simulink model "IIAFunction"  (R2024b)
settings: Solver=VariableStepAuto  StartTime=0.0  StopTime=80.0  MaxStep=0.01  RelTol=1e-3
values from neighbouring files (symbols this model uses):
  a = 2    [IIAF.m]
  Ac = 2    [IIAF.m]
  b = 2    [IIAF.m]
  Cs = 100    [IIAF.m]
  S0 = 2    [IIAF.m]
  T = 1.5    [IIAF.m]
libraries: SignalEditorBlockLib x2
settings Model: Creator=mefat  LastModifiedBy=mefat

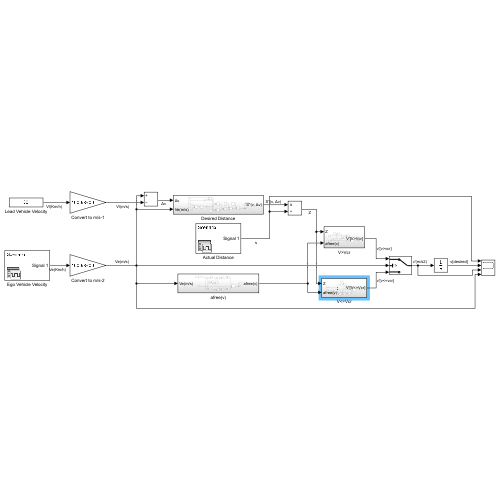
[thumbnail: Simulink's stored preview of the top-level diagram]
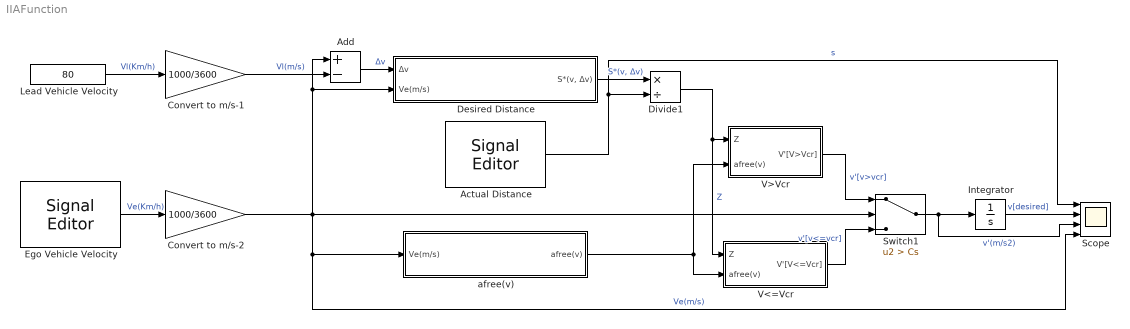
== system IIAFunction ==
  Actual Distance : SignalEditorBlockLib/Signal Editor  FileName=actual_distance.mat  ActiveScenario=Scenario  ActiveSignal=Signal 1  IsBus=off  OutputBusObjectStr=Bus: BusObject  SampleTime=0  ZeroCross=off  OutputAfterFinalValue=Setting to zero  Unit=m  PreserveSignalName=on  ApplySigPropsToAllScenarios=on  ApplySigPropsToAllSignals=off
  Add : Sum  Inputs=+-
  Convert to m/s-1 : Gain  Gain=1000/3600
  Convert to m/s-2 : Gain  Gain=1000/3600
  Desired Distance : Subsystem
  Divide1 : Product  Inputs=*/
  Ego Vehicle Velocity : SignalEditorBlockLib/Signal Editor  FileName=ego_vehicle_velocity.mat  ActiveScenario=Scenario  ActiveSignal=Signal 1  IsBus=off  OutputBusObjectStr=Bus: BusObject  SampleTime=0  ZeroCross=off  OutputAfterFinalValue=Setting to zero  Unit=m/s  PreserveSignalName=on  ApplySigPropsToAllScenarios=on  ApplySigPropsToAllSignals=off
  Integrator : Integrator
  Lead Vehicle Velocity : Constant  Value=80
  Scope : Scope  NumInputPorts=4
  Switch1 : Switch  Criteria=u2 > Threshold  Threshold=Cs  SaturateOnIntegerOverflow=off  InputSameDT=off
  V<=Vcr : Subsystem
  V>Vcr : Subsystem
  afree(v) : Subsystem
  wires:
  Convert to m/s-2/1 -> Scope/4, afree(v)/1(Ve(m/s)), Switch1/2, Add/1, Desired Distance/2(Ve(m/s))  "Ve(m/s)"
  Actual Distance/1 -> Divide1/2, Scope/1  "s"
  Ego Vehicle Velocity/1 -> Convert to m/s-2/1  "Ve(Km/h)"
  Divide1/1 -> V>Vcr/1(Z), V<=Vcr/1(Z)  "Z"
  Desired Distance/1("S*(v, Δv)") -> Divide1/1  "S*(v, Δv)"
  Lead Vehicle Velocity/1 -> Convert to m/s-1/1  "Vl(Km/h)"
  V<=Vcr/1(V'[V<=Vcr]) -> Switch1/3  "v'[v<=vcr]"
  V>Vcr/1(V'[V>Vcr]) -> Switch1/1  "v'[v>vcr]"
  Switch1/1 -> Scope/3, Integrator/1  "v'(m/s2)"
  afree(v)/1(afree(v)) -> V<=Vcr/2(afree(v)), V>Vcr/2(afree(v))
  Integrator/1 -> Scope/2  "v[desired]"
  Add/1 -> Desired Distance/1(Δv)  "Δv"
  Convert to m/s-1/1 -> Add/2  "Vl(m/s)"

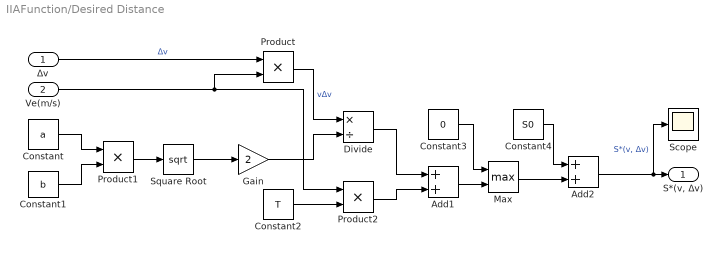
== system IIAFunction/Desired Distance ==
  Δv : Inport
  Ve(m/s) : Inport  Port=2
  Add1 : Sum
  Add2 : Sum
  Constant : Constant  Value=a
  Constant1 : Constant  Value=b
  Constant2 : Constant  Value=T
  Constant3 : Constant  Value=0
  Constant4 : Constant  Value=S0
  Divide : Product  Inputs=*/
  Gain : Gain  Gain=2
  Max : MinMax  Function=max  Inputs=2
  Product : Product
  Product1 : Product
  Product2 : Product
  Scope : Scope
  Square Root : Sqrt
  "S*(v, Δv)" : Outport
  wires:
  Constant/1 -> Product1/1
  Constant2/1 -> Product2/2
  Constant1/1 -> Product1/2
  Square Root/1 -> Gain/1
  Product1/1 -> Square Root/1
  Product2/1 -> Add1/2
  Gain/1 -> Divide/2
  Max/1 -> Add2/2
  Add1/1 -> Max/2
  Add2/1 -> Scope/1, "S*(v, Δv)"/1  "S*(v, Δv)"
  Δv/1 -> Product/1  "Δv"
  Constant4/1 -> Add2/1
  Divide/1 -> Add1/1
  Ve(m/s)/1 -> Product/2, Product2/1
  Constant3/1 -> Max/1
  Product/1 -> Divide/1  "vΔv"

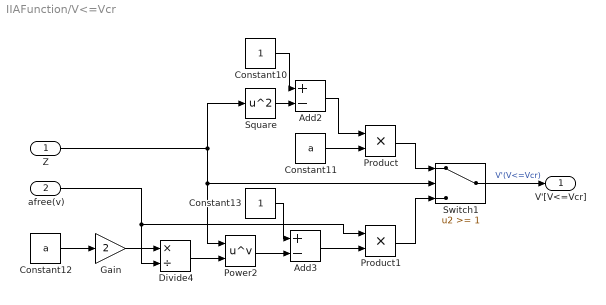
== system IIAFunction/V<=Vcr ==
  Z : Inport
  afree(v) : Inport  Port=2
  Add2 : Sum  Inputs=+-
  Add3 : Sum  Inputs=+-
  Constant10 : Constant
  Constant11 : Constant  Value=a
  Constant12 : Constant  Value=a
  Constant13 : Constant
  Divide4 : Product  Inputs=*/
  Gain : Gain  Gain=2
  Power2 : Math  Operator=pow
  Product : Product
  Product1 : Product
  Square : Math  Operator=square
  Switch1 : Switch  Threshold=1  SaturateOnIntegerOverflow=off  InputSameDT=off
  V'[V<=Vcr] : Outport
  wires:
  Constant13/1 -> Add3/1
  afree(v)/1 -> Product1/1, Divide4/2
  Switch1/1 -> V'[V<=Vcr]/1  "V'(V<=Vcr)"
  Constant10/1 -> Add2/1
  Power2/1 -> Add3/2
  Add3/1 -> Product1/2
  Product/1 -> Switch1/1
  Divide4/1 -> Power2/2
  Square/1 -> Add2/2
  Constant12/1 -> Gain/1
  Z/1 -> Power2/1, Switch1/2, Square/1
  Gain/1 -> Divide4/1
  Add2/1 -> Product/1
  Constant11/1 -> Product/2
  Product1/1 -> Switch1/3

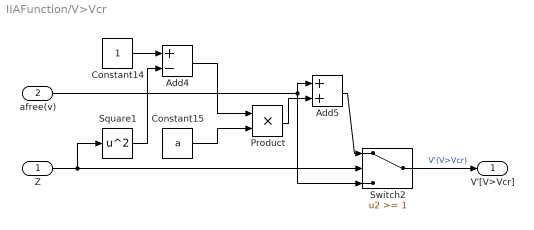
== system IIAFunction/V>Vcr ==
  Z : Inport
  afree(v) : Inport  Port=2
  Add4 : Sum  Inputs=+-
  Add5 : Sum
  Constant14 : Constant
  Constant15 : Constant  Value=a
  Product : Product
  Square1 : Math  Operator=square
  Switch2 : Switch  Threshold=1  SaturateOnIntegerOverflow=off  InputSameDT=off
  V'[V>Vcr] : Outport
  wires:
  Product/1 -> Add5/2
  Add5/1 -> Switch2/1
  Z/1 -> Switch2/2, Square1/1
  afree(v)/1 -> Add5/1, Switch2/3
  Add4/1 -> Product/1
  Constant14/1 -> Add4/1
  Square1/1 -> Add4/2
  Constant15/1 -> Product/2
  Switch2/1 -> V'[V>Vcr]/1  "V'(V>Vcr)"

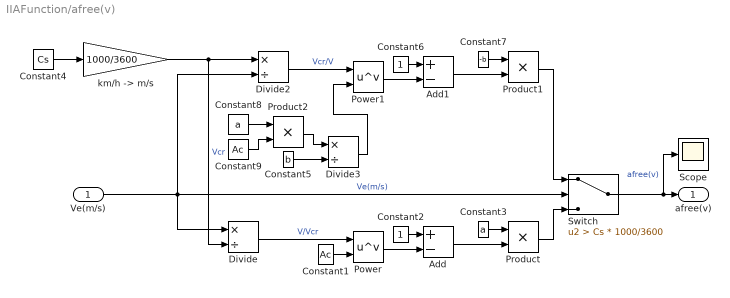
== system IIAFunction/afree(v) ==
  Ve(m/s) : Inport
  Add : Sum  Inputs=+-
  Add1 : Sum  Inputs=+-
  Constant1 : Constant  Value=Ac
  Constant2 : Constant
  Constant3 : Constant  Value=a
  Constant4 : Constant  Value=Cs
  Constant5 : Constant  Value=b
  Constant6 : Constant
  Constant7 : Constant  Value=-b
  Constant8 : Constant  Value=a
  Constant9 : Constant  Value=Ac
  Divide : Product  Inputs=*/
  Divide2 : Product  Inputs=*/
  Divide3 : Product  Inputs=*/
  Power : Math  Operator=pow
  Power1 : Math  Operator=pow
  Product : Product
  Product1 : Product
  Product2 : Product
  Scope : Scope
  Switch : Switch  Criteria=u2 > Threshold  Threshold=Cs * 1000/3600  SaturateOnIntegerOverflow=off  InputSameDT=off
  "km/h -> m/s" : Gain  Gain=1000/3600
  afree(v) : Outport
  wires:
  Product1/1 -> Switch/1
  Product/1 -> Switch/3
  Divide3/1 -> Power1/2
  Divide2/1 -> Power1/1  "Vcr/V"
  Constant2/1 -> Add/1
  Power/1 -> Add/2
  Constant3/1 -> Product/1
  Switch/1 -> Scope/1, afree(v)/1  "afree(v)"
  Add/1 -> Product/2
  Constant7/1 -> Product1/1
  Add1/1 -> Product1/2
  Constant5/1 -> Divide3/2
  Power1/1 -> Add1/2
  Constant6/1 -> Add1/1
  "km/h -> m/s"/1 -> Divide2/1, Divide/2  "Vcr"
  Divide/1 -> Power/1  "V/Vcr"
  Constant1/1 -> Power/2
  Constant4/1 -> "km/h -> m/s"/1
  Product2/1 -> Divide3/1
  Constant8/1 -> Product2/1
  Constant9/1 -> Product2/2
  Ve(m/s)/1 -> Divide2/2, Divide/1, Switch/2  "Ve(m/s)"
